simulink model "PFC_69C_03_06_V01_3Phase_3_2KW"  (R2022b)
settings: Solver=FixedStepAuto  StartTime=0.0  StopTime=Inf  RelTol=1e-3  EnableMultiTasking=on
model workspace (MAT data in the model file):
  ADC_Gain = 1241.21212121
  DAC_Gain = 0.000805860805861
  Inductor_Current_Divider_Gain_Phase_A = 33.4
  Inductor_Current_Divider_Gain_Phase_B = 33.4
  Vbulk_Divider_Gain = 276.854928018
  Vin_Divider_Gain = 556.17352614
undefined symbols (not defined in the file or in its folder): GPTRIP1SEL, GPTRIP2SEL, SCI_A_Transmit, SCI_A_Transmit_Current_Suffix, SCI_A_Transmit_one_shot_Suffix, SCI_A_Transmit_Polarity_Suffix, SCI_A_Transmit_relay_Suffix, SCI_A_Transmit_Vbulk_Suffix, SCI_A_Transmit_Vin_rms_Suffix, SCI_A_Transmit_Vin_Suffix, SCI_A_Transmit_Vmid_Suffix, SCI_A_Transmit_Vp_Suffix, SCI_A_Transmit_Vpfc_Suffix, TZ1, TZ2
libraries: c280xlib x38, c2802xlib x34, simulink x17, c2000lib x1
(part 5 of 8)

== system PFC_69C_03_06_V01_3Phase_3_2KW/PWM Update @50KHz/Fixed Duty update_Phase_C/Archive ==
  Constant : Constant  Value=100
  Data Store Read : DataStoreRead  DataStoreName=Polarity_Phase_A  IndexOptions=Index vector (dialog)  Indices=1  OutputSizes=1
  Data Store Read1 : DataStoreRead  DataStoreName=Near_Zero_Bar_Phase_A  IndexOptions=Index vector (dialog)  Indices=1  OutputSizes=1
  Data Store Read2 : DataStoreRead  DataStoreName=PWM_Duty_UART  IndexOptions=Index vector (dialog)  Indices=1  OutputSizes=1
  Data Store Read5 : DataStoreRead  DataStoreName=Near_Zero_Bar_Phase_A  IndexOptions=Index vector (dialog)  Indices=1  OutputSizes=1
  Data Store Write : DataStoreWrite  DataStoreName=PWM_Duty  IndexOptions=Index vector (dialog)  Indices=1  OutputSizes=1
  If : If  IfExpression=u1 ==1
  If Action Subsystem : Subsystem  TreatAsAtomicUnit=on
  If Action Subsystem1 : Subsystem  TreatAsAtomicUnit=on
  If Action Subsystem2 : Subsystem  TreatAsAtomicUnit=on
  If Action Subsystem3 : Subsystem  TreatAsAtomicUnit=on
  If1 : If  IfExpression=u1 ==0
  Merge : Merge
  Product : Product
  Subtract : Sum  Inputs=-+
  wires:
  If/1 -> If Action Subsystem1/Action
  Data Store Read2/1 -> If Action Subsystem1/1(In1), Subtract/1, Data Store Write/1
  Merge/1 -> Product/2
  If Action Subsystem2/1(Out1) -> Merge/2
  Constant/1 -> Subtract/2
  Data Store Read/1 -> If/1
  Subtract/1 -> If Action Subsystem2/1(In1)
  Data Store Read1/1 -> Product/1
  If/2 -> If Action Subsystem2/Action
  If Action Subsystem1/1(Out1) -> Merge/1
  If1/1 -> If Action Subsystem/Action
  Data Store Read5/1 -> If1/1
  If1/2 -> If Action Subsystem3/Action

== system PFC_69C_03_06_V01_3Phase_3_2KW/PWM Update @50KHz/Fixed Duty update_Phase_C/Subsystem1 ==
  Frequency(kHz) : Inport
  Duty(%) : Inport  Port=2
  Constant1 : Constant  Value=90E6
  Divide : Product  Inputs=*/  RndMeth=Zero  SaturateOnIntegerOverflow=on
  Gain : Gain  Gain=1000
  Gain1 : Gain  Gain=1/100
  Gain2 : Gain  Gain=0.5
  Product1 : Product
  Out1 : Outport
  Out2 : Outport  Port=2
  Out3 : Outport  Port=3
  wires:
  Gain2/1 -> Out3/1
  Gain1/1 -> Product1/2
  Product1/1 -> Gain2/1, Out2/1
  Duty(%)/1 -> Gain1/1
  Divide/1 -> Out1/1, Product1/1
  Gain/1 -> Divide/2
  Constant1/1 -> Divide/1
  Frequency(kHz)/1 -> Gain/1

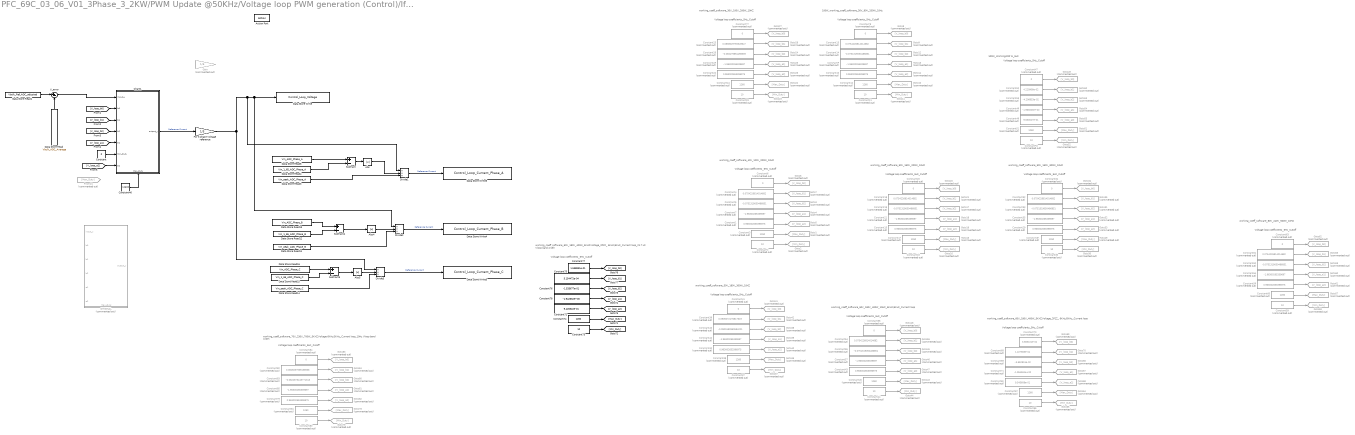
== system PFC_69C_03_06_V01_3Phase_3_2KW/PWM Update @50KHz/Voltage loop PWM generation (Control)/If Action Subsystem ==
  note: Voltage loop coefficients_5Hz_Cutoff
  note: 100W_Working/200 W_5Hz
  note: 100W_working_coeff_software_30V_90V_200W_10Hz
  note: Voltage loop coefficients_5Hz_Cutoff
  note: Voltage loop coefficients_5Hz_Cutoff
  note: working_coeff_software_30V_100V_200W_10HZ
  note: working_coeff_software_40V_120V_200W_10HZ
  note: Voltage loop coefficients_5Hz_Cutoff
  note: working_coeff_software_50V_150V_200W_10HZ
  note: Voltage loop coefficients_5Hz_Cutoff
  note: working_coeff_software_50V_150V_300W_10HZ
  note: Voltage loop coefficients_5Hz_Cutoff
  note: Voltage loop coefficients_5Hz_Cutoff
  note: working_coeff_software_50V_180V_300W_10HZ
  note: Voltage loop coefficients_5Hz_Cutoff
  note: working_coeff_software_60V_180V_400W_10HZ_6KHz/5KHz_Current loop
  note: Voltage loop coefficients_5Hz_Cutoff
  note: working_coeff_software_80V_240V_500W_10HZ
  note: Voltage loop coefficients_5Hz_Cutoff
  note: working_coeff_software_60V_180V_400W_5KHZVoltage_2P2Z_
      | 6KHz/5KHz_Current loop
  note: working_coeff_software_60V_180V_400W_5KHZVoltage_2P2Z_
      | 6KHz/5KHz_Current loop_21.7 Hz Vloop band width
  note: Voltage loop coefficients_5Hz_Cutoff
  note: Voltage loop coefficients_5Hz_Cutoff
  note: working_coeff_software_70V_230V_700W_5KHZVoltage
      | 6KHz/5KHz_Current loop_10Hz Vloop band width
  Action Port : ActionPort  ActionPortLabel=if((u1==1) & (u2==1))
  Abs : Abs  SaturateOnIntegerOverflow=off
  Abs4 : Abs  SaturateOnIntegerOverflow=off
  Abs5 : Abs  SaturateOnIntegerOverflow=off
  Chart1 : Stateflow chart  TreatAsAtomicUnit=on
      settings: PortSchema="{\"entries\":[{\"content\":{\"sides\":[{\"content\":{\"connectorIds\":[\"In2\",\"In3\",\"In4\",\"In5\",\"In7\",\"In6\",\"In8\"]},\"type\":\"ConnectorPlacement.EquallySpacedRectSide\",\"uuid\":\"98054acb-dc05-45b7-9e49-d1f1309a60af\"},{\"content\":{\"connectorIds\":[\"Out1\"],\"side\":\"RIGHT\"},\"type\":\"ConnectorPlacement.EquallySpacedRectSide\",\"uuid\":\"519c6a11-fba4-4420-9bc2-f24cec898983\"},{\"content\":{\"connectorIds\":[],\"side\":\"TOP\"},\"type\":\"ConnectorPlacement.EquallySpacedRectSide\",\"uuid\":\"37e92206-8070-4c6c-85b3-8eb12c5538cd\"},{\"content\":{\"connectorIds\":[\"In1\"],\"side\":\"BOTTOM\"},\"type\":\"ConnectorPlacement.EquallySpacedRectSide\",\"uuid\":\"a24e42b6-e88f-4c7d-a70a-f75d0d02a985\"}]},\"type\":\"ConnectorPlacement.EquallySpacedConnector\",\"uuid\":\"7d467722-ac20-43d4-98e5-7341f60d2894\"}],\"packageUris\":[\"http://schema.mathworks.com/mf0/Connector/R2020b\"],\"version\":\"1.0\"}"
  Constant : Constant  Value=0
  Constant{1,10,15,22,29,36,43,58,79} (9 alike) : Constant  Commented=on  Value=0.963002653396975
  Constant{2,11,16,23,30,37,44,50,59,66,80} (11 alike) : Constant  Commented=on  Value=10  OutDataTypeStr=double
  Constant{3,12,17,24,31,38,45,51,60,67,81} (11 alike) : Constant  Commented=on  Value=1260  OutDataTypeStr=double
  Constant{4,13,18,32,54,61} (6 alike) : Constant  Commented=on  Value=0.0754226814014682
  Constant{5,14,19,33,55,62} (6 alike) : Constant  Commented=on  Value=-0.0751319050486851
  Constant{6,8,20,27,34,41,47,56,63,84} (10 alike) : Constant  Commented=on  Value=0
  Constant{7,9,21,28,35,42,57,64,85} (9 alike) : Constant  Commented=on  Value=-1.96300265339697
  Constant25 : Constant  Commented=on  Value=0.0838029793349647
  Constant26 : Constant  Commented=on  Value=-0.083479894498539
  Constant39 : Constant  Commented=on  Value=0.0905072176817619
  Constant40 : Constant  Commented=on  Value=-0.0901582860584221
  Constant46 : Constant  Value=12600
  Constant48 : Constant  Commented=on  Value=-1.963003e+00
  Constant49 : Constant  Commented=on  Value=9.630027e-01
  Constant52 : Constant  Commented=on  Value=4.220906e-02
  Constant53 : Constant  Commented=on  Value=-4.206653e-02
  Constant65 : Constant  Commented=on  Value=9.545608e-01
  Constant68 : Constant  Commented=on  Value=1.227663e-04
  Constant69 : Constant  Commented=on  Value=-3.652824e-02
  Constant70 : Constant  Commented=on  Value=3.665101e-02
  Constant71 : Constant  Commented=on  Value=-1.954561e+00
  Constant72 : Constant  Value=9.426322e-01
  Constant73 : Constant  Value=10  OutDataTypeStr=double
  Constant74 : Constant  Value=1260  OutDataTypeStr=double
  Constant75 : Constant  Value=5.154472e-04
  Constant76 : Constant  Value=-1.533677e-01
  Constant77 : Constant  Value=1.538831e-01
  Constant78 : Constant  Value=-1.942632e+00
  Constant82 : Constant  Commented=on  Value=0.0826057939158938
  Constant83 : Constant  Commented=on  Value=-0.0822873245771313
  Data Store Read : DataStoreRead  DataStoreName=Vbulk_ADC_Average  IndexOptions=Index vector (dialog)  Indices=1  OutputSizes=1
  Data Store Read1 : DataStoreRead  DataStoreName=Vbulk_Ref_ADC_adjusted  IndexOptions=Index vector (dialog)  Indices=1  OutputSizes=1
  Data Store Read11 : DataStoreRead  DataStoreName=Vin_peak_ADC_Phase_B  IndexOptions=Index vector (dialog)  Indices=1  OutputSizes=1
  Data Store Read12 : DataStoreRead  DataStoreName=Vin_1_65_ADC_Phase_B  IndexOptions=Index vector (dialog)  Indices=1  OutputSizes=1
  Data Store Read13 : DataStoreRead  DataStoreName=Vin_ADC_Phase_B  IndexOptions=Index vector (dialog)  Indices=1  OutputSizes=1
  Data Store Read14 : DataStoreRead  DataStoreName=Vin_peak_ADC_Phase_C  IndexOptions=Index vector (dialog)  Indices=1  OutputSizes=1
  Data Store Read15 : DataStoreRead  DataStoreName=Vin_1_65_ADC_Phase_C  IndexOptions=Index vector (dialog)  Indices=1  OutputSizes=1
  Data Store Read16 : DataStoreRead  DataStoreName=Vin_ADC_Phase_C  IndexOptions=Index vector (dialog)  Indices=1  OutputSizes=1
  Data Store Read3 : DataStoreRead  DataStoreName=Vin_peak_ADC_Phase_A  IndexOptions=Index vector (dialog)  Indices=1  OutputSizes=1
  Data Store Read4 : DataStoreRead  DataStoreName=Vin_1_65_ADC_Phase_A  IndexOptions=Index vector (dialog)  Indices=1  OutputSizes=1
  Data Store Read6 : DataStoreRead  DataStoreName=Vin_ADC_Phase_A  IndexOptions=Index vector (dialog)  Indices=1  OutputSizes=1
  Data Store Write : DataStoreWrite  DataStoreName=Control_Loop_Voltage  IndexOptions=Index vector (dialog)  Indices=1  OutputSizes=1
  Data Store Write3 : DataStoreWrite  DataStoreName=Control_Loop_Current_Phase_A  IndexOptions=Index vector (dialog)  Indices=1  OutputSizes=1
  Data Store Write4 : DataStoreWrite  DataStoreName=Control_Loop_Current_Phase_B  IndexOptions=Index vector (dialog)  Indices=1  OutputSizes=1
  Data Store Write5 : DataStoreWrite  DataStoreName=Control_Loop_Current_Phase_C  IndexOptions=Index vector (dialog)  Indices=1  OutputSizes=1
  Divide1 : Product  Inputs=**/  RndMeth=Zero  SaturateOnIntegerOverflow=on
  Divide2 : Product  Inputs=**/  RndMeth=Zero  SaturateOnIntegerOverflow=on
  Divide3 : Product  Inputs=**/  RndMeth=Zero  SaturateOnIntegerOverflow=on
  For 3 phase Voltage reference : Gain  Gain=1/3
  From21 : From  Commented=on  GotoTag=Max_Duty
  Gain : Gain  Commented=on  Gain=1/6
  Goto{1,10,15,22,29,36,43,51,57,64,78} (11 alike) : Goto  Commented=on  GotoTag=Max_Duty
  Goto{2,11,16,23,30,37,44,52,58,65,79} (11 alike) : Goto  Commented=on  GotoTag=Min_Duty
  Goto{3,12,17,24,31,38,45,53,59,66,80} (11 alike) : Goto  Commented=on  GotoTag=V_loop_b2
  Goto{4,13,18,25,32,39,46,54,60,67,81} (11 alike) : Goto  Commented=on  GotoTag=V_loop_a1
  Goto{5,14,19,26,33,40,47,55,61,68,82} (11 alike) : Goto  Commented=on  GotoTag=V_loop_a2
  Goto{6,8,20,27,34,41,48..49,62,69,83} (11 alike) : Goto  Commented=on  GotoTag=V_loop_b0
  Goto{7,9,21,28,35,42,50,56,63,70,84} (11 alike) : Goto  Commented=on  GotoTag=V_loop_b1
  ORIGINAL : Stateflow chart  Commented=on  TreatAsAtomicUnit=on
      settings: PortSchema="{\"entries\":[{\"content\":{\"sides\":[{\"content\":{\"connectorIds\":[\"In2\",\"In3\",\"In4\",\"In5\",\"In6\",\"In7\"]},\"type\":\"ConnectorPlacement.EquallySpacedRectSide\",\"uuid\":\"98054acb-dc05-45b7-9e49-d1f1309a60af\"},{\"content\":{\"connectorIds\":[\"Out1\"],\"side\":\"RIGHT\"},\"type\":\"ConnectorPlacement.EquallySpacedRectSide\",\"uuid\":\"519c6a11-fba4-4420-9bc2-f24cec898983\"},{\"content\":{\"connectorIds\":[],\"side\":\"TOP\"},\"type\":\"ConnectorPlacement.EquallySpacedRectSide\",\"uuid\":\"37e92206-8070-4c6c-85b3-8eb12c5538cd\"},{\"content\":{\"connectorIds\":[\"In1\"],\"side\":\"BOTTOM\"},\"type\":\"ConnectorPlacement.EquallySpacedRectSide\",\"uuid\":\"a24e42b6-e88f-4c7d-a70a-f75d0d02a985\"}]},\"type\":\"ConnectorPlacement.EquallySpacedConnector\",\"uuid\":\"7d467722-ac20-43d4-98e5-7341f60d2894\"}],\"packageUris\":[\"http://schema.mathworks.com/mf0/Connector/R2020b\"],\"version\":\"1.0\"}"
  Subtract : Sum  Inputs=+-
  Subtract4 : Sum  Inputs=+-
  Subtract5 : Sum  Inputs=+-
  V_error : Sum  Inputs=|+-  AccumDataTypeStr=double  OutDataTypeStr=double
  wires:
  [V_loop_a2] -> Chart1/8(a2)
  Data Store Read/1 -> V_error/2
  Data Store Read1/1 -> V_error/1
  Constant52/1 -> Goto50/1
  Constant51/1 -> Goto51/1
  Constant47/1 -> Goto49/1
  Constant50/1 -> Goto52/1
  Constant49/1 -> Goto55/1
  Constant48/1 -> Goto54/1
  Data Store Read6/1 -> Subtract/1
  Data Store Read4/1 -> Subtract/2
  Subtract/1 -> Abs/1
  Abs/1 -> Divide1/2
  Data Store Read3/1 -> Divide1/3
  Divide1/1 -> Data Store Write3/1  "Reference Current"
  Data Store Read12/1 -> Subtract4/2
  Divide2/1 -> Data Store Write4/1  "Reference Current"
  Data Store Read11/1 -> Divide2/3
  Subtract4/1 -> Abs4/1
  Abs4/1 -> Divide2/2
  Data Store Read13/1 -> Subtract4/1
  Subtract5/1 -> Abs5/1
  Abs5/1 -> Divide3/2
  Data Store Read16/1 -> Subtract5/1
  Data Store Read15/1 -> Subtract5/2
  Data Store Read14/1 -> Divide3/3
  Divide3/1 -> Data Store Write5/1  "Reference Current"
  Constant53/1 -> Goto53/1
  Chart1/1(output_y) -> For 3 phase Voltage reference/1  "Reference Current"
  Constant11/1 -> Goto11/1
  Constant12/1 -> Goto10/1
  Constant10/1 -> Goto14/1
  Constant9/1 -> Goto13/1
  Constant8/1 -> Goto8/1
  Constant13/1 -> Goto9/1
  Constant14/1 -> Goto12/1
  Constant24/1 -> Goto22/1
  Constant28/1 -> Goto25/1
  Constant27/1 -> Goto27/1
  Constant23/1 -> Goto23/1
  Constant22/1 -> Goto26/1
  Constant26/1 -> Goto24/1
  Constant25/1 -> Goto28/1
  Constant1/1 -> Goto5/1
  Constant4/1 -> Goto7/1
  Constant2/1 -> Goto2/1
  Constant6/1 -> Goto6/1
  Constant7/1 -> Goto4/1
  Constant5/1 -> Goto3/1
  Constant3/1 -> Goto1/1
  Constant19/1 -> Goto17/1
  Constant15/1 -> Goto19/1
  Constant21/1 -> Goto18/1
  Constant16/1 -> Goto16/1
  Constant17/1 -> Goto15/1
  Constant20/1 -> Goto20/1
  Constant18/1 -> Goto21/1
  Constant34/1 -> Goto34/1
  Constant35/1 -> Goto32/1
  Constant31/1 -> Goto29/1
  Constant32/1 -> Goto35/1
  Constant29/1 -> Goto33/1
  Constant30/1 -> Goto30/1
  Constant33/1 -> Goto31/1
  Constant39/1 -> Goto42/1
  Constant42/1 -> Goto39/1
  Constant38/1 -> Goto36/1
  Constant37/1 -> Goto37/1
  Constant40/1 -> Goto38/1
  Constant36/1 -> Goto40/1
  Constant41/1 -> Goto41/1
  Constant55/1 -> Goto45/1
  Constant44/1 -> Goto44/1
  Constant45/1 -> Goto43/1
  Constant56/1 -> Goto48/1
  Constant57/1 -> Goto46/1
  Constant54/1 -> Goto56/1
  Constant43/1 -> Goto47/1
  Constant58/1 -> Goto61/1
  Constant63/1 -> Goto62/1
  Constant62/1 -> Goto59/1
  Constant64/1 -> Goto60/1
  Constant61/1 -> Goto63/1
  Constant59/1 -> Goto58/1
  Constant60/1 -> Goto57/1
  Constant65/1 -> Goto68/1
  Constant71/1 -> Goto67/1
  Constant68/1 -> Goto70/1
  Constant70/1 -> Goto69/1
  Constant66/1 -> Goto65/1
  Constant67/1 -> Goto64/1
  Constant69/1 -> Goto66/1
  Constant74/1 -> [Max_Duty]
  Constant76/1 -> [V_loop_b2]
  Constant77/1 -> [V_loop_b0]
  Constant75/1 -> [V_loop_b1]
  Constant73/1 -> [Min_Duty]
  Constant72/1 -> [V_loop_a2]
  Constant78/1 -> [V_loop_a1]
  V_error/1 -> Chart1/2(input_u)
  [V_loop_b0] -> Chart1/3(b0)
  [V_loop_b1] -> Chart1/4(b1)
  [V_loop_b2] -> Chart1/5(b2)
  [V_loop_a1] -> Chart1/7(a1)
  Constant/1 -> Chart1/6(Min_Duty)
  Constant46/1 -> Chart1/1(Max_Duty)
  Constant85/1 -> Goto81/1
  Constant80/1 -> Goto79/1
  Constant84/1 -> Goto83/1
  Constant83/1 -> Goto80/1
  Constant79/1 -> Goto82/1
  Constant81/1 -> Goto78/1
  Constant82/1 -> Goto84/1
  For 3 phase Voltage reference/1 -> Divide3/1, Data Store Write/1, Divide2/1, Divide1/1

== system PFC_69C_03_06_V01_3Phase_3_2KW/UART reporting @ 1Hz/Data_calculation/DataCalculation_Phase_A ==
  function : TriggerPort  TriggerType=function-call  VariantControl=(inherit)
  Data Store Read : DataStoreRead  DataStoreName=Inductor_Current_ADC_Phase_A  IndexOptions=Index vector (dialog)  Indices=1  OutputSizes=1
  Data Store Read1 : DataStoreRead  DataStoreName=Vin_ADC_Average_Phase_A  IndexOptions=Index vector (dialog)  Indices=1  OutputSizes=1
  Data Store Read3 : DataStoreRead  DataStoreName=Inductor_Current_1_65_ADC_Phase_A  IndexOptions=Index vector (dialog)  Indices=1  OutputSizes=1
  Data Store Read4 : DataStoreRead  DataStoreName=Vin_1_65_ADC_Phase_A  IndexOptions=Index vector (dialog)  Indices=1  OutputSizes=1
  Data Store Write2 : DataStoreWrite  DataStoreName=Inductor_Current_Phase_A  IndexOptions=Index vector (dialog)  Indices=1  OutputSizes=1
  Data Store Write4 : DataStoreWrite  DataStoreName=Vin_Phase_A  IndexOptions=Index vector (dialog)  Indices=1  OutputSizes=1
  Gain2 : Gain  Gain=DAC_Gain
  Gain3 : Gain  Gain=Inductor_Current_Divider_Gain_Phase_A
  Gain4 : Gain  Gain=DAC_Gain
  Gain5 : Gain  Gain=Vin_Divider_Gain
  Gain6 : Gain  Gain=100
  Subtract1 : Sum  Inputs=+-
  Subtract2 : Sum  Inputs=+-
  wires:
  Gain5/1 -> Data Store Write4/1
  Subtract2/1 -> Gain2/1
  Gain4/1 -> Gain5/1
  Subtract1/1 -> Gain4/1
  Gain6/1 -> Data Store Write2/1
  Data Store Read4/1 -> Subtract1/2
  Gain3/1 -> Gain6/1
  Data Store Read3/1 -> Subtract2/2
  Data Store Read1/1 -> Subtract1/1
  Gain2/1 -> Gain3/1
  Data Store Read/1 -> Subtract2/1

== system PFC_69C_03_06_V01_3Phase_3_2KW/UART reporting @ 1Hz/Data_calculation/DataCalculation_Phase_B ==
  function : TriggerPort  TriggerType=function-call  VariantControl=(inherit)
  Data Store Read : DataStoreRead  DataStoreName=Inductor_Current_ADC_Phase_B  IndexOptions=Index vector (dialog)  Indices=1  OutputSizes=1
  Data Store Read1 : DataStoreRead  DataStoreName=Vin_ADC_Average_Phase_B  IndexOptions=Index vector (dialog)  Indices=1  OutputSizes=1
  Data Store Read3 : DataStoreRead  DataStoreName=Inductor_Current_1_65_ADC_Phase_B  IndexOptions=Index vector (dialog)  Indices=1  OutputSizes=1
  Data Store Read4 : DataStoreRead  DataStoreName=Vin_1_65_ADC_Phase_B  IndexOptions=Index vector (dialog)  Indices=1  OutputSizes=1
  Data Store Write2 : DataStoreWrite  DataStoreName=Inductor_Current_Phase_B  IndexOptions=Index vector (dialog)  Indices=1  OutputSizes=1
  Data Store Write4 : DataStoreWrite  DataStoreName=Vin_Phase_B  IndexOptions=Index vector (dialog)  Indices=1  OutputSizes=1
  Gain2 : Gain  Gain=DAC_Gain
  Gain3 : Gain  Gain=Inductor_Current_Divider_Gain_Phase_B
  Gain4 : Gain  Gain=DAC_Gain
  Gain5 : Gain  Gain=Vin_Divider_Gain
  Gain6 : Gain  Gain=100
  Subtract1 : Sum  Inputs=+-
  Subtract2 : Sum  Inputs=+-
  wires:
  Gain5/1 -> Data Store Write4/1
  Subtract2/1 -> Gain2/1
  Gain4/1 -> Gain5/1
  Subtract1/1 -> Gain4/1
  Gain6/1 -> Data Store Write2/1
  Data Store Read4/1 -> Subtract1/2
  Gain3/1 -> Gain6/1
  Data Store Read3/1 -> Subtract2/2
  Data Store Read1/1 -> Subtract1/1
  Gain2/1 -> Gain3/1
  Data Store Read/1 -> Subtract2/1

== system PFC_69C_03_06_V01_3Phase_3_2KW/UART reporting @ 1Hz/Data_calculation/DataCalculation_Phase_C ==
  function : TriggerPort  TriggerType=function-call  VariantControl=(inherit)
  Data Store Read : DataStoreRead  DataStoreName=Inductor_Current_ADC_Phase_C  IndexOptions=Index vector (dialog)  Indices=1  OutputSizes=1
  Data Store Read1 : DataStoreRead  DataStoreName=Vin_ADC_Average_Phase_C  IndexOptions=Index vector (dialog)  Indices=1  OutputSizes=1
  Data Store Read3 : DataStoreRead  DataStoreName=Inductor_Current_1_65_ADC_Phase_C  IndexOptions=Index vector (dialog)  Indices=1  OutputSizes=1
  Data Store Read4 : DataStoreRead  DataStoreName=Vin_1_65_ADC_Phase_C  IndexOptions=Index vector (dialog)  Indices=1  OutputSizes=1
  Data Store Write2 : DataStoreWrite  DataStoreName=Inductor_Current_Phase_C  IndexOptions=Index vector (dialog)  Indices=1  OutputSizes=1
  Data Store Write4 : DataStoreWrite  DataStoreName=Vin_Phase_C  IndexOptions=Index vector (dialog)  Indices=1  OutputSizes=1
  Gain2 : Gain  Gain=DAC_Gain
  Gain3 : Gain  Gain=Inductor_Current_Divider_Gain_Phase_B
  Gain4 : Gain  Gain=DAC_Gain
  Gain5 : Gain  Gain=Vin_Divider_Gain
  Gain6 : Gain  Gain=100
  Subtract1 : Sum  Inputs=+-
  Subtract2 : Sum  Inputs=+-
  wires:
  Gain5/1 -> Data Store Write4/1
  Subtract2/1 -> Gain2/1
  Gain4/1 -> Gain5/1
  Subtract1/1 -> Gain4/1
  Gain6/1 -> Data Store Write2/1
  Data Store Read4/1 -> Subtract1/2
  Gain3/1 -> Gain6/1
  Data Store Read3/1 -> Subtract2/2
  Data Store Read1/1 -> Subtract1/1
  Gain2/1 -> Gain3/1
  Data Store Read/1 -> Subtract2/1

== system PFC_69C_03_06_V01_3Phase_3_2KW/UART reporting @ 1Hz/Data_calculation/Vbulk&Vmid ==
  function : TriggerPort  TriggerType=function-call  VariantControl=(inherit)
  Data Store Read : DataStoreRead  DataStoreName=Vbulk  IndexOptions=Index vector (dialog)  Indices=1  OutputSizes=1
  Data Store Read1 : DataStoreRead  DataStoreName=Vmid_ADC  IndexOptions=Index vector (dialog)  Indices=1  OutputSizes=1
  Data Store Read2 : DataStoreRead  DataStoreName=Vbulk_ADC_Average  IndexOptions=Index vector (dialog)  Indices=1  OutputSizes=1
  Data Store Read3 : DataStoreRead  DataStoreName=Vmid_Topside  IndexOptions=Index vector (dialog)  Indices=1  OutputSizes=1
  Data Store Write1 : DataStoreWrite  DataStoreName=Vbulk  IndexOptions=Index vector (dialog)  Indices=1  OutputSizes=1
  Data Store Write2 : DataStoreWrite  DataStoreName=Vmid_Topside  IndexOptions=Index vector (dialog)  Indices=1  OutputSizes=1
  Data Store Write3 : DataStoreWrite  DataStoreName=Vmid_Bottomside  IndexOptions=Index vector (dialog)  Indices=1  OutputSizes=1
  Gain1 : Gain  Gain=DAC_Gain
  Gain2 : Gain  Gain=DAC_Gain
  Gain3 : Gain  Gain=155.47
  Gain7 : Gain  Gain=Vbulk_Divider_Gain  OutDataTypeStr=double
  Subtract : Sum  Inputs=+-
  wires:
  Gain7/1 -> Data Store Write1/1
  Gain1/1 -> Gain7/1
  Data Store Read2/1 -> Gain1/1
  Gain3/1 -> Data Store Write2/1
  Gain2/1 -> Gain3/1
  Data Store Read1/1 -> Gain2/1
  Data Store Read/1 -> Subtract/1
  Data Store Read3/1 -> Subtract/2
  Subtract/1 -> Data Store Write3/1

== system PFC_69C_03_06_V01_3Phase_3_2KW/UART reporting @ 1Hz/Phase_A/Duty_control_loop_Phase_A ==
  function : TriggerPort  TriggerType=function-call  VariantControl=(inherit)
  Data Store Read : DataStoreRead  Commented=on  DataStoreName=Vbulk_ADC_Average  IndexOptions=Index vector (dialog)  Indices=1  OutputSizes=1
  Data Store Read1 : DataStoreRead  DataStoreName=ePWM2A_CMPA_Phase_A  IndexOptions=Index vector (dialog)  Indices=1  OutputSizes=1
  Function Caller1 : FunctionCaller  FunctionPrototype=SCI_A_Transmit(u)  InputArgumentSpecifications=<Enter example>  OutputArgumentSpecifications=<Enter example>
  Function Caller2 : FunctionCaller  FunctionPrototype=SCI_A_Transmit_Polarity_Suffix()  InputArgumentSpecifications=<Enter example>  OutputArgumentSpecifications=<Enter example>
  Gain1 : Gain  Commented=on  Gain=DAC_Gain
  Gain7 : Gain  Commented=on  Gain=Vbulk_Divider_Gain
  wires:
  Data Store Read/1 -> Gain1/1
  Gain1/1 -> Gain7/1
  Data Store Read1/1 -> Function Caller1/1

== system PFC_69C_03_06_V01_3Phase_3_2KW/UART reporting @ 1Hz/Phase_A/Send Inductor_Current (A) ==
  function : TriggerPort  TriggerType=function-call  VariantControl=(inherit)
  Data Store Read : DataStoreRead  DataStoreName=Iin_rms_Phase_A  IndexOptions=Index vector (dialog)  Indices=1  OutputSizes=1
  Function Caller1 : FunctionCaller  FunctionPrototype=SCI_A_Transmit(u)  InputArgumentSpecifications=<Enter example>  OutputArgumentSpecifications=<Enter example>
  Function Caller2 : FunctionCaller  FunctionPrototype=SCI_A_Transmit_Current_Suffix()  InputArgumentSpecifications=<Enter example>  OutputArgumentSpecifications=<Enter example>
  wires:
  Data Store Read/1 -> Function Caller1/1

== system PFC_69C_03_06_V01_3Phase_3_2KW/UART reporting @ 1Hz/Phase_A/Send PFC_en_Phase_A ==
  function : TriggerPort  TriggerType=function-call  VariantControl=(inherit)
  Data Store Read : DataStoreRead  DataStoreName=PFC_en_Phase_A  IndexOptions=Index vector (dialog)  Indices=1  OutputSizes=1
  Function Caller1 : FunctionCaller  FunctionPrototype=SCI_A_Transmit(u)  InputArgumentSpecifications=<Enter example>  OutputArgumentSpecifications=<Enter example>
  Function Caller2 : FunctionCaller  FunctionPrototype=SCI_A_Transmit_Vp_Suffix()  InputArgumentSpecifications=<Enter example>  OutputArgumentSpecifications=<Enter example>
  wires:
  Data Store Read/1 -> Function Caller1/1

== system PFC_69C_03_06_V01_3Phase_3_2KW/UART reporting @ 1Hz/Phase_A/Send Vin (V) ==
  function : TriggerPort  TriggerType=function-call  VariantControl=(inherit)
  Data Store Read1 : DataStoreRead  DataStoreName=Vin_Phase_A  IndexOptions=Index vector (dialog)  Indices=1  OutputSizes=1
  Function Caller1 : FunctionCaller  FunctionPrototype=SCI_A_Transmit(u)  InputArgumentSpecifications=<Enter example>  OutputArgumentSpecifications=<Enter example>
  Function Caller2 : FunctionCaller  FunctionPrototype=SCI_A_Transmit_Vin_Suffix()  InputArgumentSpecifications=<Enter example>  OutputArgumentSpecifications=<Enter example>
  wires:
  Data Store Read1/1 -> Function Caller1/1

== system PFC_69C_03_06_V01_3Phase_3_2KW/UART reporting @ 1Hz/Phase_A/Send Vin_rms (V) ==
  function : TriggerPort  TriggerType=function-call  VariantControl=(inherit)
  Data Store Read1 : DataStoreRead  DataStoreName=Vin_rms_Phase_A  IndexOptions=Index vector (dialog)  Indices=1  OutputSizes=1
  Function Caller1 : FunctionCaller  FunctionPrototype=SCI_A_Transmit(u)  InputArgumentSpecifications=<Enter example>  OutputArgumentSpecifications=<Enter example>
  Function Caller2 : FunctionCaller  FunctionPrototype=SCI_A_Transmit_Vin_rms_Suffix()  InputArgumentSpecifications=<Enter example>  OutputArgumentSpecifications=<Enter example>
  wires:
  Data Store Read1/1 -> Function Caller1/1

== system PFC_69C_03_06_V01_3Phase_3_2KW/UART reporting @ 1Hz/Phase_A/Send control_loop_current ==
  function : TriggerPort  TriggerType=function-call  VariantControl=(inherit)
  Data Store Read1 : DataStoreRead  DataStoreName=One_Shot_Bar  IndexOptions=Index vector (dialog)  Indices=1  OutputSizes=1
  Function Caller1 : FunctionCaller  FunctionPrototype=SCI_A_Transmit(u)  InputArgumentSpecifications=<Enter example>  OutputArgumentSpecifications=<Enter example>
  Function Caller2 : FunctionCaller  FunctionPrototype=SCI_A_Transmit_Vin_rms_Suffix()  InputArgumentSpecifications=<Enter example>  OutputArgumentSpecifications=<Enter example>
  wires:
  Data Store Read1/1 -> Function Caller1/1

== system PFC_69C_03_06_V01_3Phase_3_2KW/UART reporting @ 1Hz/Phase_B/Duty_control_loop_Phase_B ==
  function : TriggerPort  TriggerType=function-call  VariantControl=(inherit)
  Data Store Read : DataStoreRead  Commented=on  DataStoreName=Vbulk_ADC_Average  IndexOptions=Index vector (dialog)  Indices=1  OutputSizes=1
  Data Store Read1 : DataStoreRead  DataStoreName=ePWM1A_CMPA_Phase_B  IndexOptions=Index vector (dialog)  Indices=1  OutputSizes=1
  Function Caller1 : FunctionCaller  FunctionPrototype=SCI_A_Transmit(u)  InputArgumentSpecifications=<Enter example>  OutputArgumentSpecifications=<Enter example>
  Function Caller2 : FunctionCaller  FunctionPrototype=SCI_A_Transmit_Polarity_Suffix()  InputArgumentSpecifications=<Enter example>  OutputArgumentSpecifications=<Enter example>
  Gain1 : Gain  Commented=on  Gain=DAC_Gain
  Gain7 : Gain  Commented=on  Gain=Vbulk_Divider_Gain
  Phase_B : Constant  Commented=on  Value=[66]  OutDataTypeStr=uint8
  SCI Transmit : c280xlib/SCI Transmit  Commented=on  sciModule=A  dataHead=''  dataTail=10  blockingMode=on  outputStatus=off
  wires:
  Data Store Read/1 -> Gain1/1
  Gain1/1 -> Gain7/1
  Data Store Read1/1 -> Function Caller1/1
  Phase_B/1 -> SCI Transmit/1

== system PFC_69C_03_06_V01_3Phase_3_2KW/UART reporting @ 1Hz/Phase_B/Send Inductor_Current (A) ==
  function : TriggerPort  TriggerType=function-call  VariantControl=(inherit)
  Data Store Read : DataStoreRead  DataStoreName=Iin_rms_Phase_B  IndexOptions=Index vector (dialog)  Indices=1  OutputSizes=1
  Function Caller1 : FunctionCaller  FunctionPrototype=SCI_A_Transmit(u)  InputArgumentSpecifications=<Enter example>  OutputArgumentSpecifications=<Enter example>
  Function Caller2 : FunctionCaller  FunctionPrototype=SCI_A_Transmit_Current_Suffix()  InputArgumentSpecifications=<Enter example>  OutputArgumentSpecifications=<Enter example>
  Phase_B : Constant  Commented=on  Value=[66]  OutDataTypeStr=uint8
  SCI Transmit : c280xlib/SCI Transmit  Commented=on  sciModule=A  dataHead=''  dataTail=10  blockingMode=on  outputStatus=off
  wires:
  Data Store Read/1 -> Function Caller1/1
  Phase_B/1 -> SCI Transmit/1

== system PFC_69C_03_06_V01_3Phase_3_2KW/UART reporting @ 1Hz/Phase_B/Send PFC_en_Phase_B ==
  function : TriggerPort  TriggerType=function-call  VariantControl=(inherit)
  Data Store Read : DataStoreRead  DataStoreName=PFC_en_Phase_B  IndexOptions=Index vector (dialog)  Indices=1  OutputSizes=1
  Function Caller1 : FunctionCaller  FunctionPrototype=SCI_A_Transmit(u)  InputArgumentSpecifications=<Enter example>  OutputArgumentSpecifications=<Enter example>
  Function Caller2 : FunctionCaller  FunctionPrototype=SCI_A_Transmit_Vp_Suffix()  InputArgumentSpecifications=<Enter example>  OutputArgumentSpecifications=<Enter example>
  Phase_B : Constant  Commented=on  Value=[66]  OutDataTypeStr=uint8
  SCI Transmit : c280xlib/SCI Transmit  Commented=on  sciModule=A  dataHead=''  dataTail=10  blockingMode=on  outputStatus=off
  wires:
  Data Store Read/1 -> Function Caller1/1
  Phase_B/1 -> SCI Transmit/1

== system PFC_69C_03_06_V01_3Phase_3_2KW/UART reporting @ 1Hz/Phase_B/Send Vin (V) ==
  function : TriggerPort  TriggerType=function-call  VariantControl=(inherit)
  Data Store Read1 : DataStoreRead  DataStoreName=Vin_Phase_B  IndexOptions=Index vector (dialog)  Indices=1  OutputSizes=1
  Function Caller1 : FunctionCaller  FunctionPrototype=SCI_A_Transmit(u)  InputArgumentSpecifications=<Enter example>  OutputArgumentSpecifications=<Enter example>
  Function Caller2 : FunctionCaller  FunctionPrototype=SCI_A_Transmit_Vin_Suffix()  InputArgumentSpecifications=<Enter example>  OutputArgumentSpecifications=<Enter example>
  Phase_B : Constant  Commented=on  Value=[66]  OutDataTypeStr=uint8
  SCI Transmit : c280xlib/SCI Transmit  Commented=on  sciModule=A  dataHead=''  dataTail=10  blockingMode=on  outputStatus=off
  wires:
  Data Store Read1/1 -> Function Caller1/1
  Phase_B/1 -> SCI Transmit/1

== system PFC_69C_03_06_V01_3Phase_3_2KW/UART reporting @ 1Hz/Phase_B/Send Vin_rms (V) ==
  function : TriggerPort  TriggerType=function-call  VariantControl=(inherit)
  Data Store Read1 : DataStoreRead  DataStoreName=Vin_rms_Phase_B  IndexOptions=Index vector (dialog)  Indices=1  OutputSizes=1
  Function Caller1 : FunctionCaller  FunctionPrototype=SCI_A_Transmit(u)  InputArgumentSpecifications=<Enter example>  OutputArgumentSpecifications=<Enter example>
  Function Caller2 : FunctionCaller  FunctionPrototype=SCI_A_Transmit_Vin_rms_Suffix()  InputArgumentSpecifications=<Enter example>  OutputArgumentSpecifications=<Enter example>
  Phase_B : Constant  Commented=on  Value=[66]  OutDataTypeStr=uint8
  SCI Transmit : c280xlib/SCI Transmit  Commented=on  sciModule=A  dataHead=''  dataTail=10  blockingMode=on  outputStatus=off
  wires:
  Data Store Read1/1 -> Function Caller1/1
  Phase_B/1 -> SCI Transmit/1

== system PFC_69C_03_06_V01_3Phase_3_2KW/UART reporting @ 1Hz/Phase_B/Send control loop current ==
  function : TriggerPort  TriggerType=function-call  VariantControl=(inherit)
  Data Store Read1 : DataStoreRead  DataStoreName=Control_Loop_Current_Phase_B  IndexOptions=Index vector (dialog)  Indices=1  OutputSizes=1
  Function Caller1 : FunctionCaller  FunctionPrototype=SCI_A_Transmit(u)  InputArgumentSpecifications=<Enter example>  OutputArgumentSpecifications=<Enter example>
  Function Caller2 : FunctionCaller  FunctionPrototype=SCI_A_Transmit_Vin_rms_Suffix()  InputArgumentSpecifications=<Enter example>  OutputArgumentSpecifications=<Enter example>
  Phase_B : Constant  Commented=on  Value=[66]  OutDataTypeStr=uint8
  SCI Transmit : c280xlib/SCI Transmit  Commented=on  sciModule=A  dataHead=''  dataTail=10  blockingMode=on  outputStatus=off
  wires:
  Data Store Read1/1 -> Function Caller1/1
  Phase_B/1 -> SCI Transmit/1

== system PFC_69C_03_06_V01_3Phase_3_2KW/UART reporting @ 1Hz/Phase_C/Duty_control_loop_Phase_C ==
  function : TriggerPort  TriggerType=function-call  VariantControl=(inherit)
  Data Store Read : DataStoreRead  Commented=on  DataStoreName=Vbulk_ADC_Average  IndexOptions=Index vector (dialog)  Indices=1  OutputSizes=1
  Data Store Read1 : DataStoreRead  DataStoreName=ePWM3A_CMPA_Phase_C  IndexOptions=Index vector (dialog)  Indices=1  OutputSizes=1
  Function Caller1 : FunctionCaller  FunctionPrototype=SCI_A_Transmit(u)  InputArgumentSpecifications=<Enter example>  OutputArgumentSpecifications=<Enter example>
  Function Caller2 : FunctionCaller  FunctionPrototype=SCI_A_Transmit_Polarity_Suffix()  InputArgumentSpecifications=<Enter example>  OutputArgumentSpecifications=<Enter example>
  Gain1 : Gain  Commented=on  Gain=DAC_Gain
  Gain7 : Gain  Commented=on  Gain=Vbulk_Divider_Gain
  Phase_C : Constant  Commented=on  Value=[67]  OutDataTypeStr=uint8
  SCI Transmit : c280xlib/SCI Transmit  Commented=on  sciModule=A  dataHead=''  dataTail=10  blockingMode=on  outputStatus=off
  wires:
  Data Store Read/1 -> Gain1/1
  Gain1/1 -> Gain7/1
  Data Store Read1/1 -> Function Caller1/1
  Phase_C/1 -> SCI Transmit/1

== system PFC_69C_03_06_V01_3Phase_3_2KW/UART reporting @ 1Hz/Phase_C/Send Inductor_Current (A) ==
  function : TriggerPort  TriggerType=function-call  VariantControl=(inherit)
  Data Store Read : DataStoreRead  DataStoreName=Iin_rms_Phase_C  IndexOptions=Index vector (dialog)  Indices=1  OutputSizes=1
  Function Caller1 : FunctionCaller  FunctionPrototype=SCI_A_Transmit(u)  InputArgumentSpecifications=<Enter example>  OutputArgumentSpecifications=<Enter example>
  Function Caller2 : FunctionCaller  FunctionPrototype=SCI_A_Transmit_Current_Suffix()  InputArgumentSpecifications=<Enter example>  OutputArgumentSpecifications=<Enter example>
  Phase_C : Constant  Commented=on  Value=[67]  OutDataTypeStr=uint8
  SCI Transmit : c280xlib/SCI Transmit  Commented=on  sciModule=A  dataHead=''  dataTail=10  blockingMode=on  outputStatus=off
  wires:
  Data Store Read/1 -> Function Caller1/1
  Phase_C/1 -> SCI Transmit/1

== system PFC_69C_03_06_V01_3Phase_3_2KW/UART reporting @ 1Hz/Phase_C/Send PFC_en_Phase_C ==
  function : TriggerPort  TriggerType=function-call  VariantControl=(inherit)
  Data Store Read : DataStoreRead  DataStoreName=PFC_en_Phase_C  IndexOptions=Index vector (dialog)  Indices=1  OutputSizes=1
  Function Caller1 : FunctionCaller  FunctionPrototype=SCI_A_Transmit(u)  InputArgumentSpecifications=<Enter example>  OutputArgumentSpecifications=<Enter example>
  Function Caller2 : FunctionCaller  FunctionPrototype=SCI_A_Transmit_Vp_Suffix()  InputArgumentSpecifications=<Enter example>  OutputArgumentSpecifications=<Enter example>
  Phase_C : Constant  Commented=on  Value=[67]  OutDataTypeStr=uint8
  SCI Transmit : c280xlib/SCI Transmit  Commented=on  sciModule=A  dataHead=''  dataTail=10  blockingMode=on  outputStatus=off
  wires:
  Data Store Read/1 -> Function Caller1/1
  Phase_C/1 -> SCI Transmit/1

== system PFC_69C_03_06_V01_3Phase_3_2KW/UART reporting @ 1Hz/Phase_C/Send Vin (V) ==
  function : TriggerPort  TriggerType=function-call  VariantControl=(inherit)
  Data Store Read1 : DataStoreRead  DataStoreName=Vin_Phase_C  IndexOptions=Index vector (dialog)  Indices=1  OutputSizes=1
  Function Caller1 : FunctionCaller  FunctionPrototype=SCI_A_Transmit(u)  InputArgumentSpecifications=<Enter example>  OutputArgumentSpecifications=<Enter example>
  Function Caller2 : FunctionCaller  FunctionPrototype=SCI_A_Transmit_Vin_Suffix()  InputArgumentSpecifications=<Enter example>  OutputArgumentSpecifications=<Enter example>
  Phase_C : Constant  Commented=on  Value=[67]  OutDataTypeStr=uint8
  SCI Transmit : c280xlib/SCI Transmit  Commented=on  sciModule=A  dataHead=''  dataTail=10  blockingMode=on  outputStatus=off
  wires:
  Data Store Read1/1 -> Function Caller1/1
  Phase_C/1 -> SCI Transmit/1

== system PFC_69C_03_06_V01_3Phase_3_2KW/UART reporting @ 1Hz/Phase_C/Send Vin_rms (V) ==
  function : TriggerPort  TriggerType=function-call  VariantControl=(inherit)
  Data Store Read1 : DataStoreRead  DataStoreName=Vin_rms_Phase_C  IndexOptions=Index vector (dialog)  Indices=1  OutputSizes=1
  Function Caller1 : FunctionCaller  FunctionPrototype=SCI_A_Transmit(u)  InputArgumentSpecifications=<Enter example>  OutputArgumentSpecifications=<Enter example>
  Function Caller2 : FunctionCaller  FunctionPrototype=SCI_A_Transmit_Vin_rms_Suffix()  InputArgumentSpecifications=<Enter example>  OutputArgumentSpecifications=<Enter example>
  Phase_C : Constant  Commented=on  Value=[67]  OutDataTypeStr=uint8
  SCI Transmit : c280xlib/SCI Transmit  Commented=on  sciModule=A  dataHead=''  dataTail=10  blockingMode=on  outputStatus=off
  wires:
  Data Store Read1/1 -> Function Caller1/1
  Phase_C/1 -> SCI Transmit/1

== system PFC_69C_03_06_V01_3Phase_3_2KW/UART reporting @ 1Hz/Phase_C/Send control loop current ==
  function : TriggerPort  TriggerType=function-call  VariantControl=(inherit)
  Data Store Read1 : DataStoreRead  DataStoreName=Control_Loop_Current_Phase_C  IndexOptions=Index vector (dialog)  Indices=1  OutputSizes=1
  Function Caller1 : FunctionCaller  FunctionPrototype=SCI_A_Transmit(u)  InputArgumentSpecifications=<Enter example>  OutputArgumentSpecifications=<Enter example>
  Function Caller2 : FunctionCaller  FunctionPrototype=SCI_A_Transmit_Vin_rms_Suffix()  InputArgumentSpecifications=<Enter example>  OutputArgumentSpecifications=<Enter example>
  Phase_C : Constant  Commented=on  Value=[67]  OutDataTypeStr=uint8
  SCI Transmit : c280xlib/SCI Transmit  Commented=on  sciModule=A  dataHead=''  dataTail=10  blockingMode=on  outputStatus=off
  wires:
  Data Store Read1/1 -> Function Caller1/1
  Phase_C/1 -> SCI Transmit/1

== system PFC_69C_03_06_V01_3Phase_3_2KW/Calibration,RMS, Fault Protection @5kHz/Fault checking/If Action Subsystem/Bulk_OVP_Latch ==
  note: Output Voltage_Latch_OVP
  note: Vbulk_OVP_Threshold initialized in Data Store Memory
  function : TriggerPort  TriggerType=function-call  VariantControl=(inherit)
  Chart2 : Stateflow chart  TreatAsAtomicUnit=on
  Data Store Read : DataStoreRead  DataStoreName=Vbulk_ADC_Average  IndexOptions=Index vector (dialog)  Indices=1  OutputSizes=1
  Data Store Read1 : DataStoreRead  DataStoreName=Vbulk_OVP_Threshold  IndexOptions=Index vector (dialog)  Indices=1  OutputSizes=1
  Data Store Write1 : DataStoreWrite  DataStoreName=One_Shot_Bar  IndexOptions=Index vector (dialog)  Indices=1  OutputSizes=1
  Gain2 : Gain  Gain=DAC_Gain
  Gain3 : Gain  Gain=Vbulk_Divider_Gain  OutDataTypeStr=double
  wires:
  Chart2/1(One_Shot_Bar) -> Data Store Write1/1
  Data Store Read1/1 -> Chart2/2(Vbulk_OVP_Threshold)
  Gain2/1 -> Gain3/1
  Data Store Read/1 -> Gain2/1
  Gain3/1 -> Chart2/1(input_Vbulk)

== system PFC_69C_03_06_V01_3Phase_3_2KW/Calibration,RMS, Fault Protection @5kHz/Fault checking/If Action Subsystem/Fault Check (Bulk UVP) ==
  function : TriggerPort  TriggerType=function-call  VariantControl=(inherit)
  Chart : Stateflow chart  TreatAsAtomicUnit=on
  Data Store Read1 : DataStoreRead  DataStoreName=Vbulk_ADC_Average  IndexOptions=Index vector (dialog)  Indices=1  OutputSizes=1
  Data Store Read2 : DataStoreRead  DataStoreName=Vbulk_Ref_ADC  IndexOptions=Index vector (dialog)  Indices=1  OutputSizes=1
  Data Store Read3 : DataStoreRead  DataStoreName=Soft_Start  IndexOptions=Index vector (dialog)  Indices=1  OutputSizes=1
  Data Store Read4 : DataStoreRead  DataStoreName=Vbulk_ADC  IndexOptions=Index vector (dialog)  Indices=1  OutputSizes=1
  Data Store Write : DataStoreWrite  DataStoreName=One_Shot_Bar  IndexOptions=Index vector (dialog)  Indices=1  OutputSizes=1
  Gain2 : Gain  Gain=DAC_Gain
  Gain3 : Gain  Gain=Vbulk_Divider_Gain  OutDataTypeStr=double
  wires:
  Data Store Read3/1 -> Chart/1(Soft_Start)
  Chart/1(Vbulk_UVP_Flag) -> Data Store Write/1
  Gain2/1 -> Gain3/1
  Data Store Read1/1 -> Gain2/1
  Gain3/1 -> Chart/4(Vbulk)
  Data Store Read2/1 -> Chart/3(Vbulk_Ref_ADC)
  Data Store Read4/1 -> Chart/2(Vbulk_ADC)

== system PFC_69C_03_06_V01_3Phase_3_2KW/Calibration,RMS, Fault Protection @5kHz/Fault checking/If Action Subsystem/Mid(Bottom side)_OVP_Latc ==
  note: Output Voltage_Latch_OVP
  note: Vbulk_OVP_Threshold initialized in Data Store Memory
  function : TriggerPort  TriggerType=function-call  VariantControl=(inherit)
  Chart2 : Stateflow chart  TreatAsAtomicUnit=on
  Data Store Read : DataStoreRead  DataStoreName=Vmid_Bottomside  IndexOptions=Index vector (dialog)  Indices=1  OutputSizes=1
  Data Store Read1 : DataStoreRead  DataStoreName=Vmid_OVP_Threshold  IndexOptions=Index vector (dialog)  Indices=1  OutputSizes=1
  Data Store Write1 : DataStoreWrite  DataStoreName=One_Shot_Bar  IndexOptions=Index vector (dialog)  Indices=1  OutputSizes=1
  wires:
  Data Store Read1/1 -> Chart2/2(Vbulk_OVP_Threshold)
  Chart2/1(One_Shot_Bar) -> Data Store Write1/1
  Data Store Read/1 -> Chart2/1(input_Vbulk)

== system PFC_69C_03_06_V01_3Phase_3_2KW/Calibration,RMS, Fault Protection @5kHz/Fault checking/If Action Subsystem/Mid(Top side)_OVP_Latch ==
  note: Output Voltage_Latch_OVP
  note: Vbulk_OVP_Threshold initialized in Data Store Memory
  function : TriggerPort  TriggerType=function-call  VariantControl=(inherit)
  Chart2 : Stateflow chart  TreatAsAtomicUnit=on
  Data Store Read : DataStoreRead  DataStoreName=Vmid_ADC_Average  IndexOptions=Index vector (dialog)  Indices=1  OutputSizes=1
  Data Store Read1 : DataStoreRead  DataStoreName=Vmid_OVP_Threshold  IndexOptions=Index vector (dialog)  Indices=1  OutputSizes=1
  Data Store Write1 : DataStoreWrite  DataStoreName=One_Shot_Bar  IndexOptions=Index vector (dialog)  Indices=1  OutputSizes=1
  Gain1 : Gain  Gain=155.47
  Gain2 : Gain  Gain=DAC_Gain
  wires:
  Chart2/1(One_Shot_Bar) -> Data Store Write1/1
  Data Store Read1/1 -> Chart2/2(Vbulk_OVP_Threshold)
  Gain2/1 -> Gain1/1
  Data Store Read/1 -> Gain2/1
  Gain1/1 -> Chart2/1(input_Vbulk)

== system PFC_69C_03_06_V01_3Phase_3_2KW/Calibration,RMS, Fault Protection @5kHz/Fault checking/If Action Subsystem/PFC_en_update_3Phase ==
  function : TriggerPort  TriggerType=function-call  VariantControl=(inherit)
  Chart : Stateflow chart  TreatAsAtomicUnit=on
  Constant : Constant  Commented=on
  Data Store Read1 : DataStoreRead  DataStoreName=PFC_en_Phase_A  IndexOptions=Index vector (dialog)  Indices=1  OutputSizes=1
  Data Store Read2 : DataStoreRead  DataStoreName=PFC_en_Phase_B  IndexOptions=Index vector (dialog)  Indices=1  OutputSizes=1
  Data Store Read4 : DataStoreRead  DataStoreName=PFC_en_Phase_C  IndexOptions=Index vector (dialog)  Indices=1  OutputSizes=1
  Data Store Write : DataStoreWrite  DataStoreName=PFC_en  IndexOptions=Index vector (dialog)  Indices=1  OutputSizes=1
  wires:
  Chart/1(PFC_en) -> Data Store Write/1
  Data Store Read1/1 -> Chart/1(PFC_en_Phase_A)
  Data Store Read2/1 -> Chart/2(PFC_en_Phase_B)
  Data Store Read4/1 -> Chart/3(PFC_en_Phase_C)

== system PFC_69C_03_06_V01_3Phase_3_2KW/Calibration,RMS, Fault Protection @5kHz/Fault checking/If Action Subsystem/PFC_en_update_Phase_A ==
  function : TriggerPort  TriggerType=function-call  VariantControl=(inherit)
  Chart : Stateflow chart  TreatAsAtomicUnit=on
  Data Store Read1 : DataStoreRead  DataStoreName=Vin_UVP_Flag_Phase_A  IndexOptions=Index vector (dialog)  Indices=1  OutputSizes=1
  Data Store Read2 : DataStoreRead  DataStoreName=Vin_OVP_Flag_Phase_A  IndexOptions=Index vector (dialog)  Indices=1  OutputSizes=1
  Data Store Read4 : DataStoreRead  DataStoreName=Iin_OCP_Flag_phase_A  IndexOptions=Index vector (dialog)  Indices=1  OutputSizes=1
  Data Store Write : DataStoreWrite  DataStoreName=PFC_en_Phase_A  IndexOptions=Index vector (dialog)  Indices=1  OutputSizes=1
  Data Store Write1 : DataStoreWrite  DataStoreName=PFC_en1  IndexOptions=Index vector (dialog)  Indices=1  OutputSizes=1
  wires:
  Chart/2(PFC_en1) -> Data Store Write1/1
  Data Store Read1/1 -> Chart/1(Vin_UVP_Flag)
  Data Store Read2/1 -> Chart/2(Vin_OVP_Flag)
  Chart/1(PFC_en) -> Data Store Write/1
  Data Store Read4/1 -> Chart/3(Iin_OCP_Flag)

== system PFC_69C_03_06_V01_3Phase_3_2KW/Calibration,RMS, Fault Protection @5kHz/Fault checking/If Action Subsystem/PFC_en_update_Phase_B ==
  function : TriggerPort  TriggerType=function-call  VariantControl=(inherit)
  Chart : Stateflow chart  TreatAsAtomicUnit=on
  Data Store Read : DataStoreRead  Commented=on  DataStoreName=counter_Relay  IndexOptions=Index vector (dialog)  Indices=1  OutputSizes=1
  Data Store Read1 : DataStoreRead  DataStoreName=Vin_UVP_Flag_Phase_B  IndexOptions=Index vector (dialog)  Indices=1  OutputSizes=1
  Data Store Read2 : DataStoreRead  DataStoreName=Vin_OVP_Flag_Phase_B  IndexOptions=Index vector (dialog)  Indices=1  OutputSizes=1
  Data Store Read4 : DataStoreRead  DataStoreName=Iin_OCP_Flag_phase_B  IndexOptions=Index vector (dialog)  Indices=1  OutputSizes=1
  Data Store Write : DataStoreWrite  DataStoreName=PFC_en_Phase_B  IndexOptions=Index vector (dialog)  Indices=1  OutputSizes=1
  Data Store Write1 : DataStoreWrite  DataStoreName=PFC_en1  IndexOptions=Index vector (dialog)  Indices=1  OutputSizes=1
  Data Store Write2 : DataStoreWrite  Commented=on  DataStoreName=counter_Relay  IndexOptions=Index vector (dialog)  Indices=1  OutputSizes=1
  Product : Product  Commented=on
  wires:
  Chart/2(PFC_en1) -> Data Store Write1/1
  Data Store Read1/1 -> Chart/1(Vin_UVP_Flag)
  Data Store Read/1 -> Product/2
  Product/1 -> Data Store Write2/1
  Chart/1(PFC_en) -> Product/1, Data Store Write/1
  Data Store Read2/1 -> Chart/2(Vin_OVP_Flag)
  Data Store Read4/1 -> Chart/3(Iin_OCP_Flag)

== system PFC_69C_03_06_V01_3Phase_3_2KW/Calibration,RMS, Fault Protection @5kHz/Fault checking/If Action Subsystem/PFC_en_update_Phase_C ==
  function : TriggerPort  TriggerType=function-call  VariantControl=(inherit)
  Chart : Stateflow chart  TreatAsAtomicUnit=on
  Data Store Read : DataStoreRead  Commented=on  DataStoreName=counter_Relay  IndexOptions=Index vector (dialog)  Indices=1  OutputSizes=1
  Data Store Read1 : DataStoreRead  DataStoreName=Vin_UVP_Flag_Phase_C  IndexOptions=Index vector (dialog)  Indices=1  OutputSizes=1
  Data Store Read2 : DataStoreRead  DataStoreName=Vin_OVP_Flag_Phase_C  IndexOptions=Index vector (dialog)  Indices=1  OutputSizes=1
  Data Store Read4 : DataStoreRead  DataStoreName=Iin_OCP_Flag_phase_C  IndexOptions=Index vector (dialog)  Indices=1  OutputSizes=1
  Data Store Write : DataStoreWrite  DataStoreName=PFC_en_Phase_C  IndexOptions=Index vector (dialog)  Indices=1  OutputSizes=1
  Data Store Write1 : DataStoreWrite  DataStoreName=PFC_en1  IndexOptions=Index vector (dialog)  Indices=1  OutputSizes=1
  Data Store Write2 : DataStoreWrite  Commented=on  DataStoreName=counter_Relay  IndexOptions=Index vector (dialog)  Indices=1  OutputSizes=1
  Product : Product  Commented=on
  wires:
  Chart/2(PFC_en1) -> Data Store Write1/1
  Data Store Read1/1 -> Chart/1(Vin_UVP_Flag)
  Data Store Read/1 -> Product/2
  Product/1 -> Data Store Write2/1
  Chart/1(PFC_en) -> Product/1, Data Store Write/1
  Data Store Read2/1 -> Chart/2(Vin_OVP_Flag)
  Data Store Read4/1 -> Chart/3(Iin_OCP_Flag)

== system PFC_69C_03_06_V01_3Phase_3_2KW/Calibration,RMS, Fault Protection @5kHz/Fault checking/If Action Subsystem/Phase_A_Fault ==
  function : TriggerPort  TriggerType=function-call  VariantControl=(inherit)
  "Fault Check (Input OVP)_Phase_A " : Subsystem  TreatAsAtomicUnit=on
  "Fault Check (Input UVP)_Phase_A " : Subsystem  TreatAsAtomicUnit=on
  Function-Call Generator : simulink/Ports & Subsystems/Function-Call Generator  sample_time=-1  numberOfIterations=1  DisallowWideOutput=off
  Function-Call Split : FunctionCallSplit  IconShape=distinctive  NumOutputPorts=3  OutputPortLayout=default
  Input current_OCP_Phase_A : Subsystem  TreatAsAtomicUnit=on
  wires:
  Function-Call Generator/1 -> Function-Call Split/1
  Function-Call Split/1 -> "Fault Check (Input UVP)_Phase_A "/Trigger
  Function-Call Split/2 -> "Fault Check (Input OVP)_Phase_A "/Trigger
  Function-Call Split/3 -> Input current_OCP_Phase_A/Trigger

== system PFC_69C_03_06_V01_3Phase_3_2KW/Calibration,RMS, Fault Protection @5kHz/Fault checking/If Action Subsystem/Phase_B_Fault ==
  function : TriggerPort  TriggerType=function-call  VariantControl=(inherit)
  Fault Check (Input OVP)_Phase_B : Subsystem  TreatAsAtomicUnit=on
  Fault Check (Input UVP)_Phase_B : Subsystem  TreatAsAtomicUnit=on
  Function-Call Generator : simulink/Ports & Subsystems/Function-Call Generator  sample_time=-1  numberOfIterations=1  DisallowWideOutput=off
  Function-Call Split : FunctionCallSplit  IconShape=distinctive  NumOutputPorts=3  OutputPortLayout=default
  Input current_OCP_Phase_B : Subsystem  TreatAsAtomicUnit=on
  wires:
  Function-Call Generator/1 -> Function-Call Split/1
  Function-Call Split/1 -> Fault Check (Input UVP)_Phase_B/Trigger
  Function-Call Split/2 -> Fault Check (Input OVP)_Phase_B/Trigger
  Function-Call Split/3 -> Input current_OCP_Phase_B/Trigger
